simulink subsystem "APC_1045MR"  (R2024a)
settings: Solver=VariableStepAuto  StartTime=0.0  StopTime=10.0  RelTol=1e-3
settings Model: Creator=UASG  LastModifiedBy=UASG

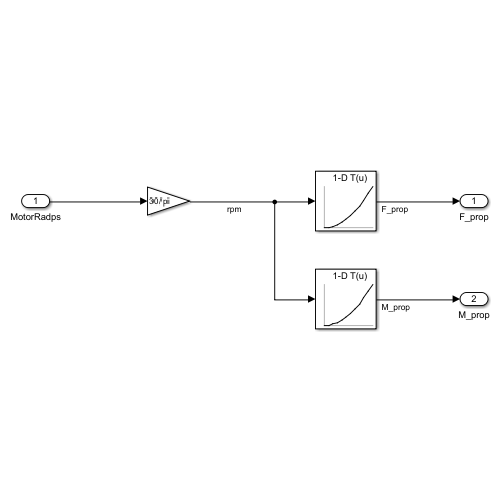
[thumbnail: Simulink's stored preview of the top-level diagram]
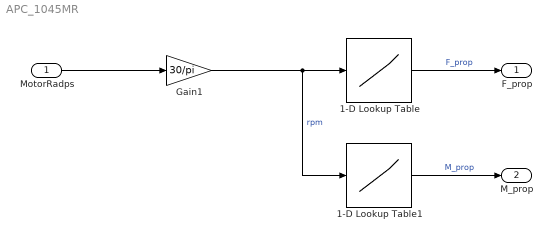
== system APC_1045MR ==
  MotorRadps : Inport
  1-D Lookup Table : Lookup_n-D  NumberOfTableDimensions=1  BreakpointsForDimension1=[0:1000:11000]  Table=[0, 0.150,0.603,1.359,2.422,3.792,5.473,7.470,9.788,12.431,15.407,18.724]  InternalRulePriority=Speed  RndMeth=Simplest
  1-D Lookup Table1 : Lookup_n-D  NumberOfTableDimensions=1  BreakpointsForDimension1=[0:1000:11000]  Table=[0,0.003,0.010,0.021,0.037,0.057,0.081,0.110,0.142,0.179,0.221,0.268]  InternalRulePriority=Speed  RndMeth=Simplest
  Gain1 : Gain  Gain=30/pi
  F_prop : Outport
  M_prop : Outport  Port=2
  wires:
  1-D Lookup Table/1 -> F_prop/1  "F_prop"
  1-D Lookup Table1/1 -> M_prop/1  "M_prop"
  Gain1/1 -> 1-D Lookup Table1/1, 1-D Lookup Table/1  "rpm"
  MotorRadps/1 -> Gain1/1
